simulink model "lqr_nl"  (R2024b)
settings: Solver=VariableStepAuto  StartTime=0.0  StopTime=params.simtime  RelTol=1e-3
values from neighbouring files (symbols this model uses):
  params = parameters()    [lqr_compare.m]    (also in lqr_main_isolated.m; lqr_pil.m)
undefined symbols (not defined in the file or in its folder): nl_model
settings Model: Creator=ben83  LastModifiedBy=ben
settings RTWCC: GPUComputeCapability=3.5

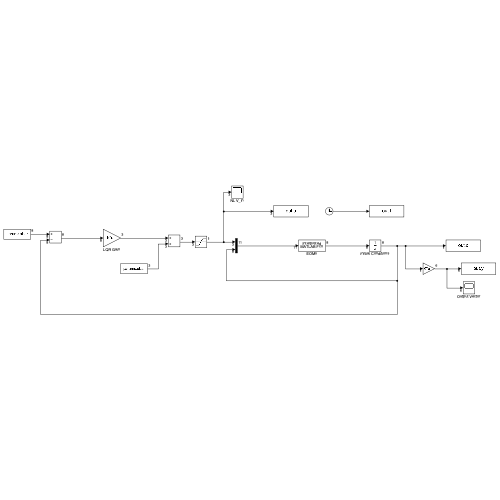
[thumbnail: Simulink's stored preview of the top-level diagram]
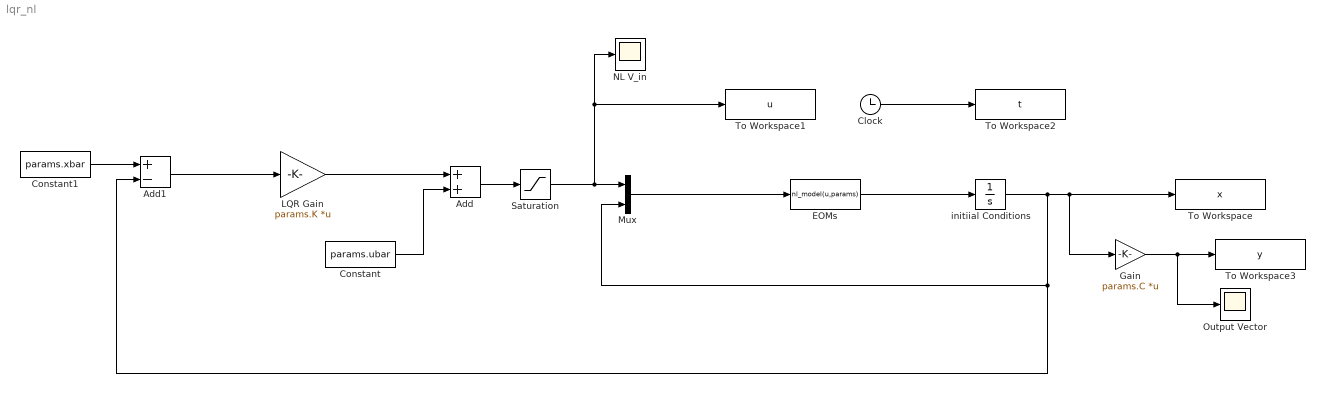
== system lqr_nl ==
  Add : Sum
  Add1 : Sum  Inputs=+-
  Clock : Clock
  Constant : Constant  Value=params.ubar
  Constant1 : Constant  Value=params.xbar
  EOMs : MATLABFcn  MATLABFcn=nl_model(u,params)  OutputDimensions=8
  Gain : Gain  Gain=params.C  Multiplication=Matrix(K*u)
  LQR Gain : Gain  Gain=params.K  Multiplication=Matrix(K*u)
  Mux : Mux  Inputs=2
  NL V_in : Scope
  Output Vector : Scope
  Saturation : Saturate  UpperLimit=11.1  LowerLimit=-11.1
  To Workspace : ToWorkspace  VariableName=x  SampleTime=-1
  To Workspace1 : ToWorkspace  VariableName=u  SampleTime=-1
  To Workspace2 : ToWorkspace  VariableName=t  SampleTime=-1
  To Workspace3 : ToWorkspace  VariableName=y  SampleTime=-1
  initiial Conditions : Integrator  InitialCondition=params.ic
  wires:
  EOMs/1 -> initiial Conditions/1
  Mux/1 -> EOMs/1
  Clock/1 -> To Workspace2/1
  Add/1 -> Saturation/1
  initiial Conditions/1 -> Mux/2, Add1/2, Gain/1, To Workspace/1
  LQR Gain/1 -> Add/1
  Constant/1 -> Add/2
  Add1/1 -> LQR Gain/1
  Constant1/1 -> Add1/1
  Gain/1 -> Output Vector/1, To Workspace3/1
  Saturation/1 -> NL V_in/1, To Workspace1/1, Mux/1
